simulink model "GPS"  (R2018a)
settings: Solver=FixedStepAuto  StartTime=0.0  StopTime=3600*12  FixedStep=0.001  RelTol=1e-3
settings Model: Creator=David  LastModifiedBy=David

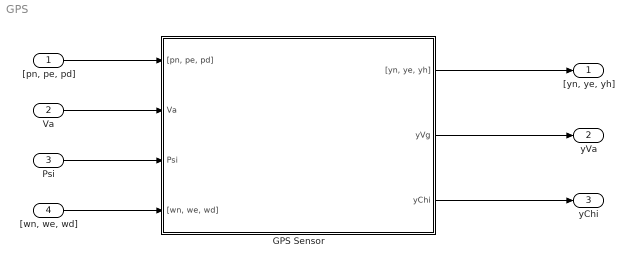
== system GPS ==
  "[pn, pe, pd]" : Inport
  Va : Inport  Port=2
  Psi : Inport  Port=3
  "[wn, we, wd]" : Inport  Port=4
  GPS Sensor : Subsystem  mask{SampleTime=0.001, GPSNStdDev=0.21, OneOverkGPSN=1100, GPSEStdDev=0.21, OneOverkGPSE=1100, GPSAltStdDev=0.4, OneOverkGPSAlt=1100, GPSVStdDev=0.2}
      mask prompts: SampleTime "GPS Sample Time (s)"; GPSNStdDev "GPS North Std Dev (m)"; OneOverkGPSN "GPS North Time Constant (s)"; GPSEStdDev "GPS East Std Dev (m)"; OneOverkGPSE "GPS East Time Constant (s)"; GPSAltStdDev "GPS Altitude Std Dev (m)"; OneOverkGPSAlt "GPS Altitude Time Constant (s)"; GPSVStdDev "GPS Velocity Std Dev (m/s)"
      mask DialogControl DescGroupVar Prompt: GPS Sensor Model
      mask DialogControl DescTextVar Prompt: GPS Sensor Model Making use of a Gauss-Markov process for noise modelling
      mask DialogControl Container4 Prompt: System Characteristics
      mask DialogControl Container5 Prompt: Noise Characteristics
      mask Display:
      | image('PiksiMulti_GPS.jpg')
      | 
      | color('green')
      | 
      | port_label('input', 1, '[p_N, p_E, p_D] (m)', 'texMode', 'On')
      | port_label('input', 2, 'V_a (m/s)', 'texMode', 'On')
      | port_label('input', 3, '\psi (rad)', 'texMode', 'On')
      | port_label('input', 4, '[w_N, w_E, w_D] (m/s)', 'texMode', 'On')
      | 
      | port_label('output', 1, '[y_{GPS_N}, y_{GPS_E}, y_{GPS_h}] (m)', 'texMode', 'On')
      | port_label('output', 2, 'y_{GPS_{Vg}} (m/s)', 'texMode', 'On')
      | port_label('output', 3, 'y_{GPS_{\chi}} (rad)', 'texMode', 'On')
  "[yn, ye, yh]" : Outport
  yVa : Outport  Port=2
  yChi : Outport  Port=3
  wires:
  "[pn, pe, pd]"/1 -> GPS Sensor/1("[pn, pe, pd]")
  GPS Sensor/1("[yn, ye, yh]") -> "[yn, ye, yh]"/1
  Va/1 -> GPS Sensor/2(Va)
  Psi/1 -> GPS Sensor/3(Psi)
  "[wn, we, wd]"/1 -> GPS Sensor/4("[wn, we, wd]")
  GPS Sensor/2(yVg) -> yVa/1
  GPS Sensor/3(yChi) -> yChi/1

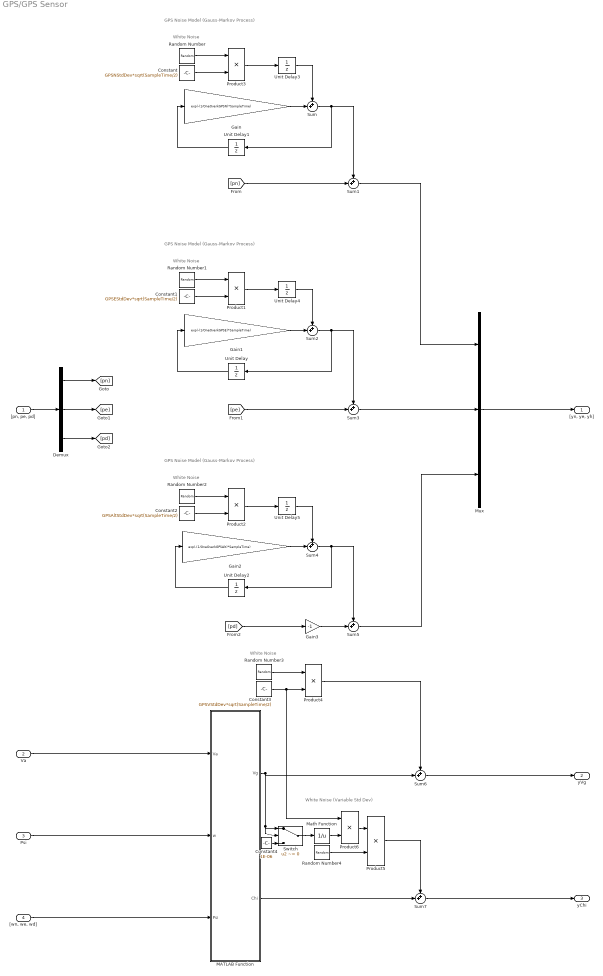
== system GPS/GPS Sensor ==
  note: GPS Noise Model (Gauss-Markov Process)
  note: White Noise
  note: White Noise
  note: GPS Noise Model (Gauss-Markov Process)
  note: White Noise
  note: GPS Noise Model (Gauss-Markov Process)
  note: White Noise
  note: White Noise (Variable Std Dev)
  "[pn, pe, pd]" : Inport
  Va : Inport  Port=2
  Psi : Inport  Port=3
  "[wn, we, wd]" : Inport  Port=4
  Constant : Constant  Value=GPSNStdDev*sqrt(SampleTime/2)
  Constant1 : Constant  Value=GPSEStdDev*sqrt(SampleTime/2)
  Constant2 : Constant  Value=GPSAltStdDev*sqrt(SampleTime/2)
  Constant3 : Constant  Value=GPSVStdDev*sqrt(SampleTime/2)
  Constant4 : Constant  Value=1E-06
  Demux : Demux  Outputs=3
  Gain : Gain  Gain=exp(-(1/OneOverkGPSN)*SampleTime)
  Gain1 : Gain  Gain=exp(-(1/OneOverkGPSE)*SampleTime)
  Gain2 : Gain  Gain=exp(-(1/OneOverkGPSAlt)*SampleTime)
  Gain3 : Gain  Gain=-1
  MATLAB Function : MATLAB Function  TreatAsAtomicUnit=on
  Math Function : Math  Operator=reciprocal  SaturateOnIntegerOverflow=on
  Mux : Mux  Inputs=3
  Product{1..6} (6 alike) : Product
  Random Number{,1..4} (5 alike) : RandomNumber  SampleTime=SampleTime
  Sum{,1..7} (8 alike) : Sum  Inputs=++|
  Switch : Switch  Criteria=u2 ~= 0
  Unit Delay{,1..5} (6 alike) : UnitDelay  SampleTime=SampleTime
  "[yn, ye, yh]" : Outport
  yVg : Outport  Port=2
  yChi : Outport  Port=3
  wires:
  Constant1/1 -> Product1/2
  [pe] -> Sum3/2
  Gain1/1 -> Sum2/2
  Unit Delay1/1 -> Gain/1
  Sum/1 -> Unit Delay1/1, Sum1/1
  Demux/3 -> [pd]
  Constant/1 -> Product3/2
  Sum2/1 -> Unit Delay/1, Sum3/1
  Unit Delay2/1 -> Gain2/1
  Constant2/1 -> Product2/2
  Sum4/1 -> Unit Delay2/1, Sum5/1
  Unit Delay/1 -> Gain1/1
  Sum3/1 -> Mux/2
  Random Number/1 -> Product3/1
  Random Number1/1 -> Product1/1
  Gain/1 -> Sum/2
  Sum1/1 -> Mux/1
  [pn] -> Sum1/2
  Mux/1 -> "[yn, ye, yh]"/1
  Gain2/1 -> Sum4/2
  Random Number2/1 -> Product2/1
  Demux/2 -> [pe]
  Sum5/1 -> Mux/3
  [pd] -> Gain3/1
  Gain3/1 -> Sum5/2
  "[pn, pe, pd]"/1 -> Demux/1
  Demux/1 -> [pn]
  Product2/1 -> Unit Delay5/1
  Product1/1 -> Unit Delay4/1
  Product3/1 -> Unit Delay3/1
  Unit Delay3/1 -> Sum/1
  Unit Delay4/1 -> Sum2/1
  Unit Delay5/1 -> Sum4/1
  "[wn, we, wd]"/1 -> MATLAB Function/3(Psi)
  Psi/1 -> MATLAB Function/2(w)
  Va/1 -> MATLAB Function/1(Va)
  Constant3/1 -> Product6/1, Product4/2
  Random Number3/1 -> Product4/1
  Product4/1 -> Sum6/1
  MATLAB Function/1(Vg) -> Sum6/2, Switch/1, Switch/2
  Random Number4/1 -> Product5/2
  Sum6/1 -> yVg/1
  Sum7/1 -> yChi/1
  Math Function/1 -> Product6/2
  Product6/1 -> Product5/1
  Product5/1 -> Sum7/1
  MATLAB Function/2(Chi) -> Sum7/2
  Switch/1 -> Math Function/1
  Constant4/1 -> Switch/3

== matlab function GPS/GPS Sensor/MATLAB Function ==
  data: Va input; Vg output; w input size=[3, 1]; Psi input; Chi output
function [Vg, Chi] = fcn(Va, w, Psi)

    wn = w(1);
    we = w(2);

    Vg = sqrt( (Va*cos(Psi) + wn)^2 + (Va*sin(Psi) + we)^2 );
    Chi = atan2( (Va*sin(Psi) + we) , (Va*cos(Psi) + wn) );
